simulink model "ClosedLoopSystemAccVar1"  (R2024b)
settings: Solver=FixedStepDiscrete  StartTime=0.0  StopTime=300  MaxStep=0.001  RelTol=1e-5
values from neighbouring files (symbols this model uses):
  A : value not decoded    [eomParameters.sldd]
  B : value not decoded    [eomParameters.sldd]
  b = 0.1    [eomParameters.sldd]
  C : value not decoded    [eomParameters.sldd]
  D : value not decoded    [eomParameters.sldd]
  d : value not decoded    [eomParameters.sldd]
  E : value not decoded    [eomParameters.sldd]
  F : value not decoded    [eomParameters.sldd]
  H : value not decoded    [eomParameters.sldd]
  I : value not decoded    [eomParameters.sldd]
  K : value not decoded    [eomParameters.sldd]
  L_1 : value not decoded    [eomParameters.sldd]
  mu = 0.4    [eomParameters.sldd]
  mu_r = 0.001    [eomParameters.sldd]
undefined symbols (not defined in the file or in its folder): DiscIntNeverNeededParam
libraries: slpidlib x1, simulink x1
settings Model: DataDictionary=eomParameters.sldd  Creator=nilgunozbulbul  LastModifiedBy=nilgunozbulbul
settings SolverCC: InitialStep=0.001

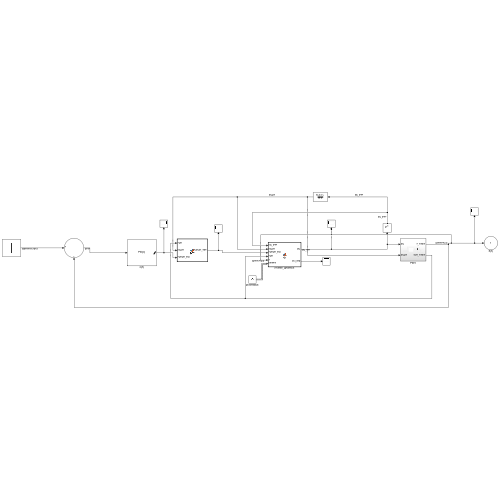
[thumbnail: Simulink's stored preview of the top-level diagram]
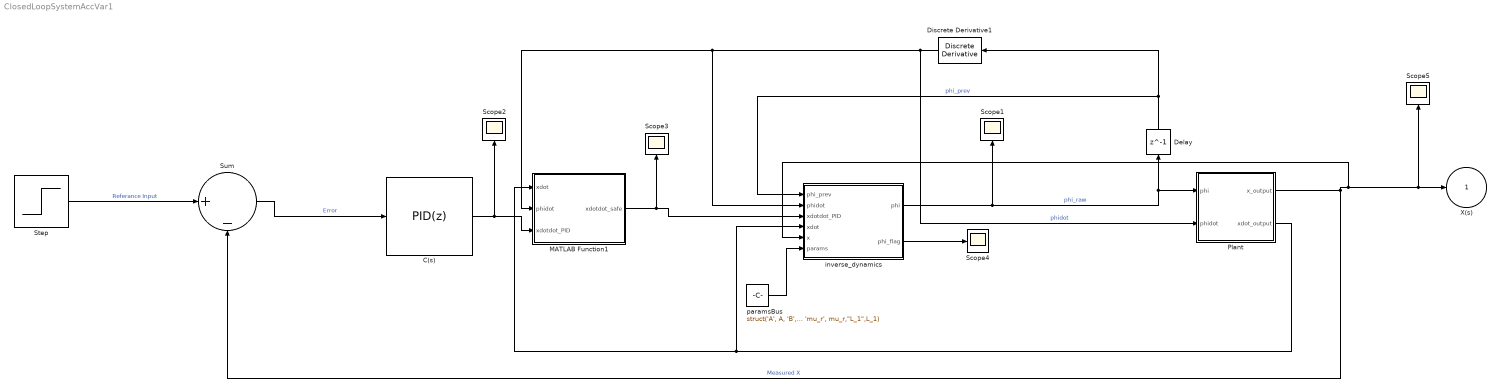
== system ClosedLoopSystemAccVar1 ==
  C(s) : slpidlib/PID Controller  Controller=PID  Form=Parallel  TimeDomain=Discrete-time  UseExternalTs=off  SampleTime=0.05  IntegratorMethod=Forward Euler  FilterMethod=Forward Euler  ControllerParametersSource=internal  P=1  I=1  UseKiTs=off  D=1  UseExternalDerivativeSource=off  N=100  UseFilter=on  TunerSelectOption=Frequency Response Based  InitialConditionSource=internal  InitialConditionForIntegrator=0  InitialConditionForFilter=0  DifferentiatorICPrevScaledInput=0  ExternalReset=none  TrackingMode=off  Kt=1  LimitOutput=on  SatLimitsSource=internal  UpperSaturationLimit=8  LowerSaturationLimit=-8  LinearizeAsGain=off  AntiWindupMode=back-calculation  Kb=1  LimitIntegrator=on  UpperIntegratorSaturationLimit=0.1  LowerIntegratorSaturationLimit=-0.1  POutMin=[]  POutMax=[]  IOutMin=[]  IOutMax=[]  DOutMin=[]  DOutMax=[]  NOutMin=[]  NOutMax=[]  SumOutMin=[]  SumOutMax=[]  SaturationOutMin=[]  SaturationOutMax=[]  PParamMin=[]  PParamMax=[]  IParamMin=[]  IParamMax=[]  DParamMin=[]  DParamMax=[]  NParamMin=[]  NParamMax=[]  KbParamMin=[]  KbParamMax=[]  KtParamMin=[]  KtParamMax=[]  KbOutMin=[]  KbOutMax=[]  KtOutMin=[]  KtOutMax=[]  IntegratorOutMin=[]  IntegratorOutMax=[]  FilterOutMin=[]  FilterOutMax=[]  SumI1OutMin=[]  SumI1OutMax=[]  SumI2OutMin=[]  SumI2OutMax=[]  SumI3OutMin=[]  SumI3OutMax=[]  SumI4OutMin=[]  SumI4OutMax=[]  SumDOutMin=[]  SumDOutMax=[]  DifferentiatorOutMin=[]  DifferentiatorOutMax=[]  FilterDiffOutCoefMin=[]  FilterDiffOutCoefMax=[]  ReciprocalOutMin=[]  ReciprocalOutMax=[]  SumDenOutMin=[]  SumDenOutMax=[]  SumNumOutMin=[]  SumNumOutMax=[]  DivideOutMin=[]  DivideOutMax=[]  UdiffTsProdOutMin=[]  UdiffTsProdOutMax=[]  NTsProdOutMin=[]  NTsProdOutMax=[]  UintegralTsProdOutMin=[]  UintegralTsProdOutMax=[]  UngainTsProdOutMin=[]  UngainTsProdOutMax=[]  ClampingZeroOutDataTypeStr=Inherit: Inherit via back propagation  ClampingZeroOutMin=[]  ClampingZeroOutMax=[]  FilterDenConstantOutDataTypeStr=Inherit: Inherit via back propagation  FilterDenConstantOutMin=[]  FilterDenConstantOutMax=[]  PCopyOutDataTypeStr=Inherit: Inherit via back propagation  PCopyOutMin=[]  PCopyOutMax=[]  NCopyOutDataTypeStr=Inherit: Inherit via back propagation  NCopyOutMin=[]  NCopyOutMax=[]  IntegratorContinuousStateAttributes=''  IntegratorStateMustResolveToSignalObject=off  IntegratorRTWStateStorageClass=Auto  FilterContinuousStateAttributes=''  FilterStateMustResolveToSignalObject=off  FilterRTWStateStorageClass=Auto  ParallelPVariant=InternalParameters  IdealPVariant=Disabled  IVariant=InternalParameters  DVariant=InternalParameters  IntegratorVariant=Discrete  SatVariant=Enabled  AWVariant=BackCalculation  PCopyVariant=Disabled  TRVariant=Disabled  FdbkBlocksVariant=Forward  IdealPFdbkVariant=Disabled  SatFdbkVariant=Disabled  DerivativeFilterVariant=ForwardEulerFilter  NVariant=InternalParameters  NCopyVariant=Disabled  FilterICVariant=InternalICsFilter  IntegratorICVariant=InternalICs  ExternalResetVariant=Disabled  TRSumVariant=Passthrough  SumFdbkVariant=Disabled  SumVariant=Sum_PID  TsampFilterVariant=InternalTs  TsampNgainVariant=Passthrough  TsampIntegralVariant=Disabled_SignalSpec  ExternalSaturationOutDataTypeStr=Inherit: Same as second input  DerivativeSourceVariant=ErrorSignal  PreIntVariant=InternalPreInt
      settings: LibrarySourceBlock=simulink/Discrete/Discrete PID Controller
  Delay : Delay  DelayLength=1  InitialCondition=0  SampleTime=0.05
  Discrete Derivative1 : simulink/Discrete/Discrete Derivative  gainval=1.0  ICPrevScaledInput=0.0  OutMin=[]  OutMax=[]  OutDataType=fixdt(1, 16)  OutScaling=2^-10  DoSatur=off
  MATLAB Function1 : MATLAB Function  TreatAsAtomicUnit=on
  Plant : Subsystem
  Scope{1..5} (5 alike) : Scope
  Step : Step  Time=0  After=0.05  SampleTime=0.05
  Sum : Sum  Inputs=|+-
  inverse_dynamics : MATLAB Function  TreatAsAtomicUnit=on
  paramsBus : Constant  Value="struct('A', A, 'B', B, 'C', C, 'D', D, 'E', E, 'F', F, 'H', H, 'I', I, 'K', K, 'b', b, 'd', d, 'mu', mu, 'mu_r', mu_r,\"L_1\",L_1)"  OutDataTypeStr=Bus: paramsBus
  X(s) : Outport
  wires:
  Plant/1(x_output) -> Scope5/1, X(s)/1, inverse_dynamics/5(x), Sum/2  "Measured X"
  Delay/1 -> inverse_dynamics/1(phi_prev), Discrete Derivative1/1  "phi_prev"
  inverse_dynamics/2(phi_flag) -> Scope4/1
  paramsBus/1 -> inverse_dynamics/6(params)
  Discrete Derivative1/1 -> Plant/2(phidot), MATLAB Function1/2(phidot), inverse_dynamics/2(phidot)  "phidot"
  Plant/2(xdot_output) -> MATLAB Function1/1(xdot), inverse_dynamics/4(xdot)
  Sum/1 -> C(s)/1  "Error"
  inverse_dynamics/1(phi) -> Scope1/1, Delay/1, Plant/1(phi)  "phi_raw"
  C(s)/1 -> Scope2/1, MATLAB Function1/3(xdotdot_PID)
  MATLAB Function1/1(xdotdot_safe) -> Scope3/1, inverse_dynamics/3(xdotdot_PID)
  Step/1 -> Sum/1  "Referance Input"

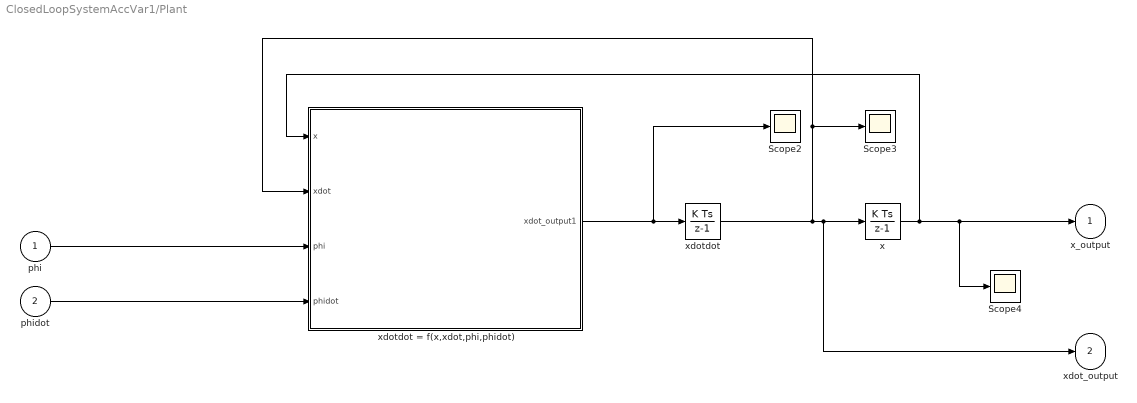
== system ClosedLoopSystemAccVar1/Plant ==
  phi : Inport
  phidot : Inport  Port=2
  Scope2 : Scope
  Scope3 : Scope
  Scope4 : Scope
  x : DiscreteIntegrator  InitialCondition=0.05  SampleTime=0.05  UpperSaturationLimit=+100  LowerSaturationLimit=-100  ICPrevOutput=DiscIntNeverNeededParam  ICPrevScaledInput=DiscIntNeverNeededParam
  xdotdot : DiscreteIntegrator  InitialCondition=0.1  SampleTime=0.05  UpperSaturationLimit=+100  LowerSaturationLimit=-100  ICPrevOutput=DiscIntNeverNeededParam  ICPrevScaledInput=DiscIntNeverNeededParam
  xdotdot = f(x,xdot,phi,phidot) : Subsystem
  x_output : Outport
  xdot_output : Outport  Port=2
  wires:
  x/1 -> xdotdot = f(x,xdot,phi,phidot)/1(x), Scope4/1, x_output/1
  xdotdot = f(x,xdot,phi,phidot)/1(xdot_output1) -> xdotdot/1, Scope2/1
  phi/1 -> xdotdot = f(x,xdot,phi,phidot)/3(phi)
  xdotdot/1 -> Scope3/1, xdotdot = f(x,xdot,phi,phidot)/2(xdot), xdot_output/1, x/1
  phidot/1 -> xdotdot = f(x,xdot,phi,phidot)/4(phidot)

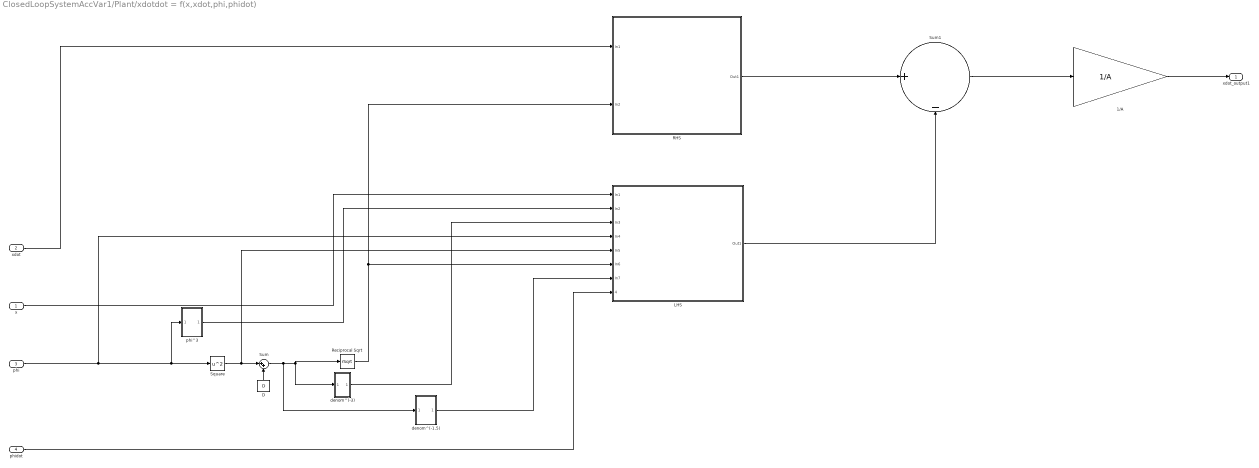
== system ClosedLoopSystemAccVar1/Plant/xdotdot = f(x,xdot,phi,phidot) ==
  x : Inport
  xdot : Inport  Port=2
  phi : Inport  Port=3
  phidot : Inport  Port=4
  1/A : Gain  Gain=1/A
  D : Constant  Value=D
  LHS : Subsystem
  RHS : Subsystem
  Reciprocal Sqrt : Sqrt  Operator=rSqrt
  Square : Math  Operator=square
  Sum : Sum  Inputs=|++
  Sum1 : Sum  Inputs=|+-
  denom^(-1.5) : Subsystem
  denom^(-3) : Subsystem
  phi^3 : Subsystem
  xdot_output1 : Outport
  wires:
  phi/1 -> LHS/4(In4), Square/1, phi^3/1(In1)
  Square/1 -> LHS/5(In5), Sum/1
  D/1 -> Sum/2
  Reciprocal Sqrt/1 -> LHS/6(In6), RHS/2(In2)
  Sum/1 -> Reciprocal Sqrt/1, denom^(-3)/1(In1), denom^(-1.5)/1(In1)
  xdot/1 -> RHS/1(In1)
  x/1 -> LHS/1(In1)
  phi^3/1(Out1) -> LHS/2(In2)
  denom^(-3)/1(Out1) -> LHS/3(In3)
  denom^(-1.5)/1(Out1) -> LHS/7(In7)
  phidot/1 -> LHS/8(4)
  RHS/1(Out1) -> Sum1/1
  LHS/1(Out1) -> Sum1/2
  Sum1/1 -> 1/A/1
  1/A/1 -> xdot_output1/1

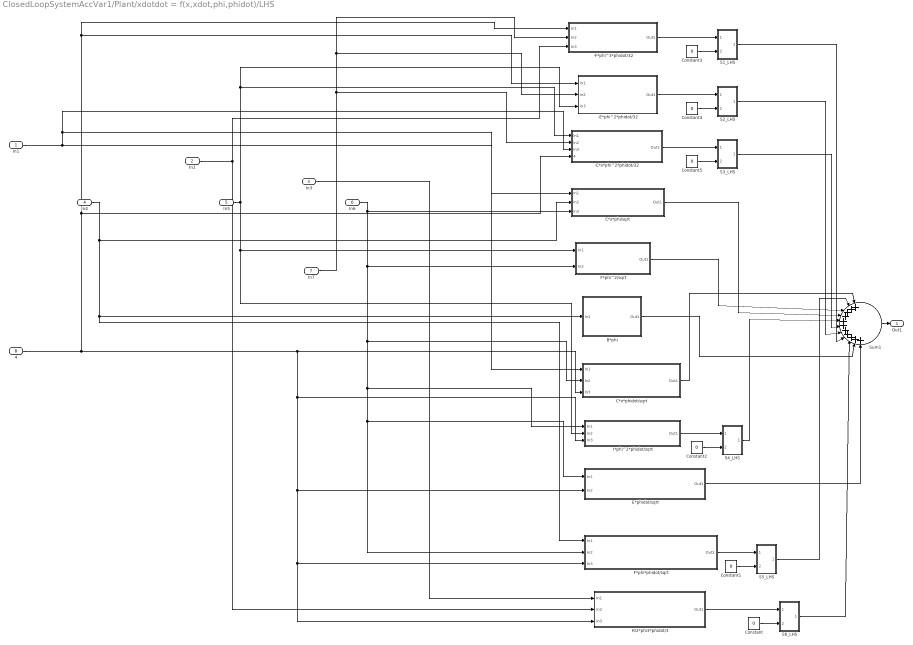
== system ClosedLoopSystemAccVar1/Plant/xdotdot = f(x,xdot,phi,phidot)/LHS ==
  In1 : Inport
  In2 : Inport  Port=2
  In3 : Inport  Port=3
  In4 : Inport  Port=4
  In5 : Inport  Port=5
  In6 : Inport  Port=6
  In7 : Inport  Port=7
  4 : Inport  Port=8
  -C*x*phi^2*phidot/32 : Subsystem
  -E*phi^2*phidot/32 : Subsystem
  -F*phi^3*phidot/32 : Subsystem
  B*phi : Subsystem
  C*x*phi/sqrt : Subsystem
  C*x*phidot/sqrt : Subsystem
  Constant{,1..5} (6 alike) : Constant  Value=0
  E*phidot/sqrt : Subsystem
  F*phi*phidot/sqrt : Subsystem
  F*phi^2/sqrt : Subsystem
  H/2*phi3*phidot/3 : Subsystem
  I*phi^2*phidot/sqrt : Subsystem
  S1_LHS : Subsystem
  S2_LHS : Subsystem
  S3_LHS : Subsystem
  S4_LHS : Subsystem
  S5_LHS : Subsystem
  S6_LHS : Subsystem
  Sum1 : Sum  Inputs=|+++++++++++
  Out1 : Outport
  wires:
  C*x*phi/sqrt/1(Out1) -> Sum1/4
  F*phi^2/sqrt/1(Out1) -> Sum1/3
  C*x*phidot/sqrt/1(Out1) -> Sum1/1
  Sum1/1 -> Out1/1
  In7/1 -> -F*phi^3*phidot/32/2(In2), -E*phi^2*phidot/32/2(In2), -C*x*phi^2*phidot/32/2(In2)
  In5/1 -> F*phi^2/sqrt/1(In1), I*phi^2*phidot/sqrt/2(In2), -E*phi^2*phidot/32/3(In3), -C*x*phi^2*phidot/32/1(In1)
  E*phidot/sqrt/1(Out1) -> Sum1/11
  B*phi/1(Out1) -> Sum1/10
  In2/1 -> H/2*phi3*phidot/3/2(In2), -F*phi^3*phidot/32/3(In3)
  In1/1 -> C*x*phidot/sqrt/1(In1), -C*x*phi^2*phidot/32/3(In3), C*x*phi/sqrt/1(In1)
  In3/1 -> H/2*phi3*phidot/3/1(In1)
  In4/1 -> C*x*phi/sqrt/2(In2), F*phi*phidot/sqrt/1(In1), B*phi/1(In1)
  In6/1 -> F*phi^2/sqrt/2(In2), I*phi^2*phidot/sqrt/1(In1), E*phidot/sqrt/1(In1), F*phi*phidot/sqrt/2(In2), C*x*phidot/sqrt/2(In2), C*x*phi/sqrt/3(In3)
  4/1 -> -F*phi^3*phidot/32/1(In1), -E*phi^2*phidot/32/1(In1), -C*x*phi^2*phidot/32/4(4), F*phi*phidot/sqrt/3(In3), H/2*phi3*phidot/3/3(In3), E*phidot/sqrt/2(In2), I*phi^2*phidot/sqrt/3(In3), C*x*phidot/sqrt/3(In3)
  Constant/1 -> S6_LHS/2(In2)
  H/2*phi3*phidot/3/1(Out1) -> S6_LHS/1(In1)
  S6_LHS/1(Out1) -> Sum1/9
  Constant1/1 -> S5_LHS/2(In2)
  F*phi*phidot/sqrt/1(Out1) -> S5_LHS/1(In1)
  S5_LHS/1(Out1) -> Sum1/2
  Constant2/1 -> S4_LHS/2(In2)
  I*phi^2*phidot/sqrt/1(Out1) -> S4_LHS/1(In1)
  S4_LHS/1(Out1) -> Sum1/5
  Constant3/1 -> S1_LHS/2(In2)
  Constant4/1 -> S2_LHS/2(In2)
  Constant5/1 -> S3_LHS/2(In2)
  -F*phi^3*phidot/32/1(Out1) -> S1_LHS/1(In1)
  -E*phi^2*phidot/32/1(Out1) -> S2_LHS/1(In1)
  -C*x*phi^2*phidot/32/1(Out1) -> S3_LHS/1(In1)
  S3_LHS/1(Out1) -> Sum1/6
  S2_LHS/1(Out1) -> Sum1/7
  S1_LHS/1(Out1) -> Sum1/8

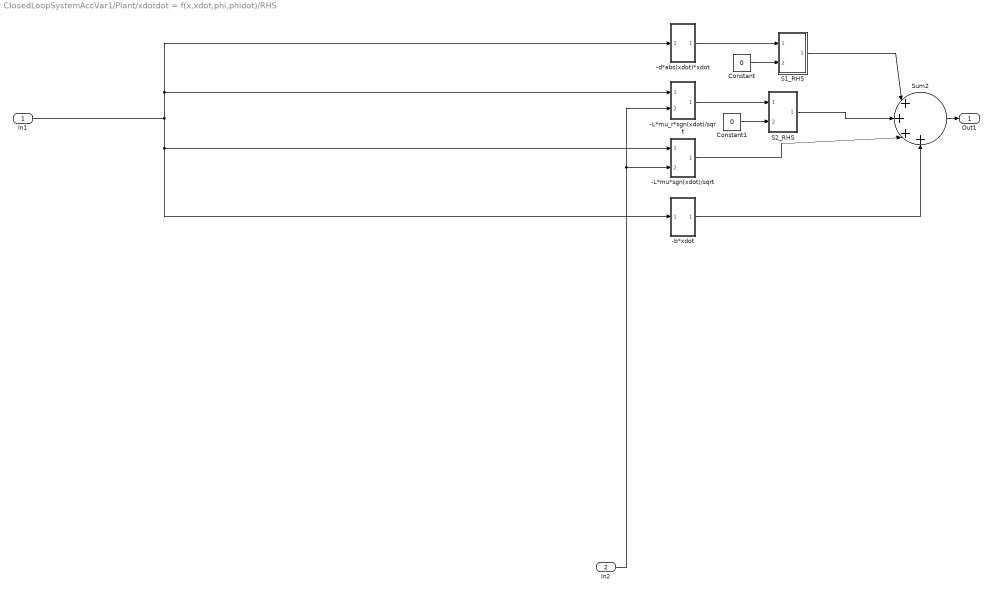
== system ClosedLoopSystemAccVar1/Plant/xdotdot = f(x,xdot,phi,phidot)/RHS ==
  In1 : Inport
  In2 : Inport  Port=2
  -L*mu*sgn(xdot)/sqrt : Subsystem
  -L*mu_r*sgn(xdot)/sqrt : Subsystem
  -b*xdot : Subsystem
  -d*abs(xdot)*xdot : Subsystem
  Constant : Constant  Value=0
  Constant1 : Constant  Value=0
  S1_RHS : Subsystem
  S2_RHS : Subsystem
  Sum2 : Sum  Inputs=|++++
  Out1 : Outport
  wires:
  Sum2/1 -> Out1/1
  -L*mu*sgn(xdot)/sqrt/1(Out1) -> Sum2/3
  -b*xdot/1(Out1) -> Sum2/4
  In1/1 -> -d*abs(xdot)*xdot/1(In1), -L*mu_r*sgn(xdot)/sqrt/1(In1), -b*xdot/1(In1), -L*mu*sgn(xdot)/sqrt/1(In1)
  In2/1 -> -L*mu_r*sgn(xdot)/sqrt/2(In2), -L*mu*sgn(xdot)/sqrt/2(In2)
  Constant/1 -> S1_RHS/2(In2)
  -d*abs(xdot)*xdot/1(Out1) -> S1_RHS/1(In1)
  S1_RHS/1(Out1) -> Sum2/1
  Constant1/1 -> S2_RHS/2(In2)
  -L*mu_r*sgn(xdot)/sqrt/1(Out1) -> S2_RHS/1(In1)
  S2_RHS/1(Out1) -> Sum2/2

== system ClosedLoopSystemAccVar1/Plant/xdotdot = f(x,xdot,phi,phidot)/denom^(-1.5) ==
  In1 : Inport
  3/2 : Constant  Value=-1.5
  Power1 : Math  Operator=pow
  Out1 : Outport
  wires:
  In1/1 -> Power1/1
  Power1/1 -> Out1/1
  3/2/1 -> Power1/2

== system ClosedLoopSystemAccVar1/Plant/xdotdot = f(x,xdot,phi,phidot)/denom^(-3) ==
  In1 : Inport
  3 : Constant  Value=-3
  Power2 : Math  Operator=pow
  Out1 : Outport
  wires:
  Power2/1 -> Out1/1
  In1/1 -> Power2/1
  3/1 -> Power2/2

== system ClosedLoopSystemAccVar1/Plant/xdotdot = f(x,xdot,phi,phidot)/phi^3 ==
  In1 : Inport
  3_ : Constant  Value=3
  Power3 : Math  Operator=pow
  Out1 : Outport
  wires:
  Power3/1 -> Out1/1
  In1/1 -> Power3/1
  3_/1 -> Power3/2

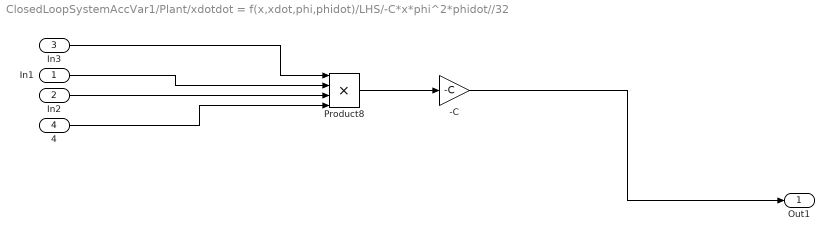
== system ClosedLoopSystemAccVar1/Plant/xdotdot = f(x,xdot,phi,phidot)/LHS/-C*x*phi^2*phidot//32 ==
  In1 : Inport
  In2 : Inport  Port=2
  In3 : Inport  Port=3
  4 : Inport  Port=4
  -C : Gain  Gain=-C
  Product8 : Product  Inputs=4
  Out1 : Outport
  wires:
  -C/1 -> Out1/1
  In2/1 -> Product8/3
  In3/1 -> Product8/1
  In1/1 -> Product8/2
  Product8/1 -> -C/1
  4/1 -> Product8/4

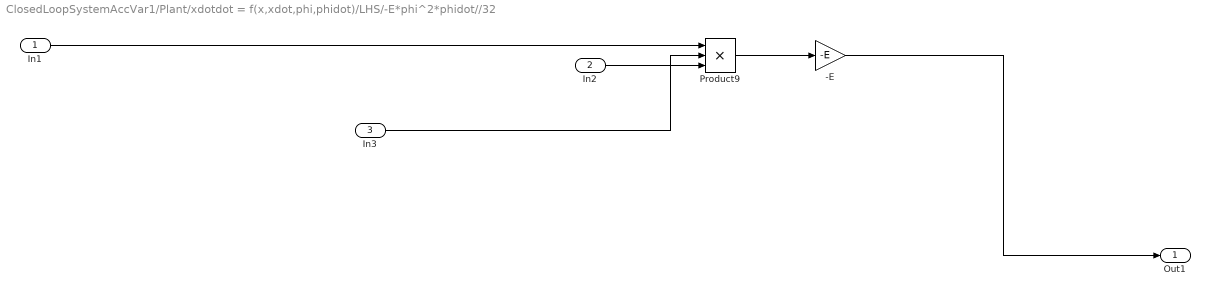
== system ClosedLoopSystemAccVar1/Plant/xdotdot = f(x,xdot,phi,phidot)/LHS/-E*phi^2*phidot//32 ==
  In1 : Inport
  In2 : Inport  Port=2
  In3 : Inport  Port=3
  -E : Gain  Gain=-E
  Product9 : Product  Inputs=3
  Out1 : Outport
  wires:
  -E/1 -> Out1/1
  In2/1 -> Product9/3
  In1/1 -> Product9/1
  In3/1 -> Product9/2
  Product9/1 -> -E/1

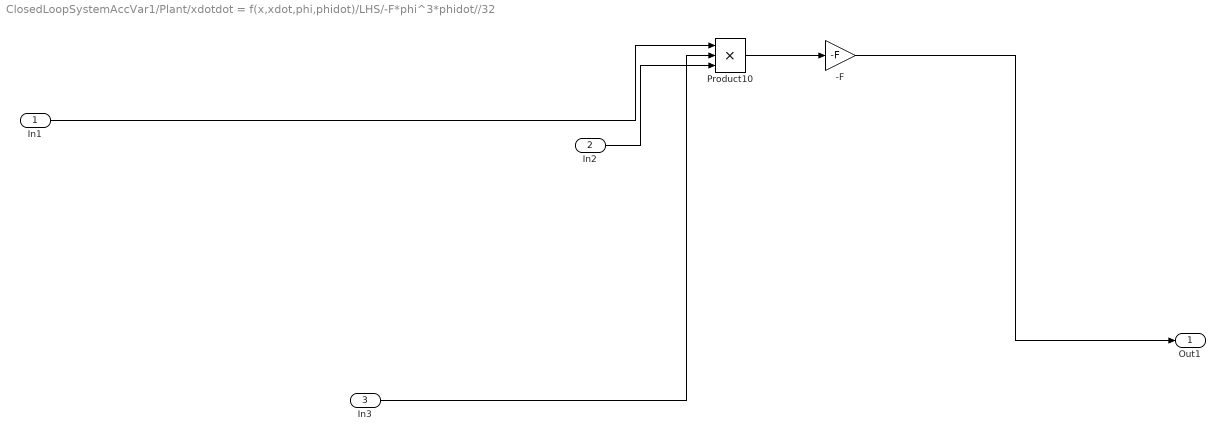
== system ClosedLoopSystemAccVar1/Plant/xdotdot = f(x,xdot,phi,phidot)/LHS/-F*phi^3*phidot//32 ==
  In1 : Inport
  In2 : Inport  Port=2
  In3 : Inport  Port=3
  -F : Gain  Gain=-F
  Product10 : Product  Inputs=3
  Out1 : Outport
  wires:
  In3/1 -> Product10/2
  -F/1 -> Out1/1
  In2/1 -> Product10/3
  In1/1 -> Product10/1
  Product10/1 -> -F/1

== system ClosedLoopSystemAccVar1/Plant/xdotdot = f(x,xdot,phi,phidot)/LHS/B*phi ==
  In1 : Inport
  B : Gain  Gain=B
  Out1 : Outport
  wires:
  In1/1 -> B/1
  B/1 -> Out1/1

== system ClosedLoopSystemAccVar1/Plant/xdotdot = f(x,xdot,phi,phidot)/LHS/C*x*phi//sqrt ==
  In1 : Inport
  In2 : Inport  Port=2
  In3 : Inport  Port=3
  C : Gain  Gain=C
  Product3 : Product  Inputs=3
  Out1 : Outport
  wires:
  In1/1 -> Product3/2
  In3/1 -> Product3/3
  C/1 -> Out1/1
  In2/1 -> Product3/1
  Product3/1 -> C/1

== system ClosedLoopSystemAccVar1/Plant/xdotdot = f(x,xdot,phi,phidot)/LHS/C*x*phidot//sqrt ==
  In1 : Inport
  In2 : Inport  Port=2
  In3 : Inport  Port=3
  C : Gain  Gain=C
  Product : Product  Inputs=3
  Out1 : Outport
  wires:
  In3/1 -> Product/3
  In1/1 -> Product/1
  In2/1 -> Product/2
  C/1 -> Out1/1
  Product/1 -> C/1

== system ClosedLoopSystemAccVar1/Plant/xdotdot = f(x,xdot,phi,phidot)/LHS/E*phidot//sqrt ==
  In1 : Inport
  In2 : Inport  Port=2
  E : Gain  Gain=E
  Product1 : Product
  Out1 : Outport
  wires:
  In2/1 -> Product1/2
  E/1 -> Out1/1
  In1/1 -> Product1/1
  Product1/1 -> E/1

== system ClosedLoopSystemAccVar1/Plant/xdotdot = f(x,xdot,phi,phidot)/LHS/F*phi*phidot//sqrt ==
  In1 : Inport
  In2 : Inport  Port=2
  In3 : Inport  Port=3
  F : Gain  Gain=F
  Product2 : Product  Inputs=3
  Out1 : Outport
  wires:
  F/1 -> Out1/1
  In2/1 -> Product2/2
  In3/1 -> Product2/1
  In1/1 -> Product2/3
  Product2/1 -> F/1

== system ClosedLoopSystemAccVar1/Plant/xdotdot = f(x,xdot,phi,phidot)/LHS/F*phi^2//sqrt ==
  In1 : Inport
  In2 : Inport  Port=2
  F : Gain  Gain=F
  Product4 : Product
  Out1 : Outport
  wires:
  F/1 -> Out1/1
  In1/1 -> Product4/2
  In2/1 -> Product4/1
  Product4/1 -> F/1

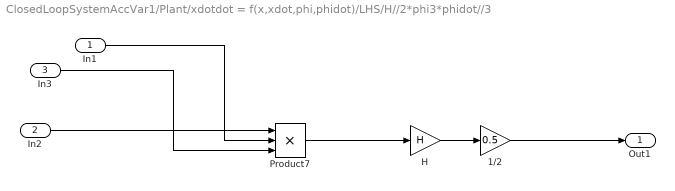
== system ClosedLoopSystemAccVar1/Plant/xdotdot = f(x,xdot,phi,phidot)/LHS/H//2*phi3*phidot//3 ==
  In1 : Inport
  In2 : Inport  Port=2
  In3 : Inport  Port=3
  1/2 : Gain  Gain=0.5
  H : Gain  Gain=H
  Product7 : Product  Inputs=3
  Out1 : Outport
  wires:
  In2/1 -> Product7/1
  In1/1 -> Product7/2
  In3/1 -> Product7/3
  Product7/1 -> H/1
  1/2/1 -> Out1/1
  H/1 -> 1/2/1

== system ClosedLoopSystemAccVar1/Plant/xdotdot = f(x,xdot,phi,phidot)/LHS/I*phi^2*phidot//sqrt ==
  In1 : Inport
  In2 : Inport  Port=2
  In3 : Inport  Port=3
  I : Gain  Gain=I
  Product11 : Product  Inputs=3
  Out1 : Outport
  wires:
  I/1 -> Out1/1
  In3/1 -> Product11/3
  In2/1 -> Product11/2
  In1/1 -> Product11/1
  Product11/1 -> I/1

== system ClosedLoopSystemAccVar1/Plant/xdotdot = f(x,xdot,phi,phidot)/LHS/S1_LHS ==
  In1 : Inport
  In2 : Inport  Port=2
  Constant1 : Constant  Value=0
  Switch : Switch  Criteria=u2 ~= 0  SaturateOnIntegerOverflow=off  InputSameDT=off
  Out1 : Outport
  wires:
  In1/1 -> Switch/1
  Switch/1 -> Out1/1
  In2/1 -> Switch/2
  Constant1/1 -> Switch/3

== system ClosedLoopSystemAccVar1/Plant/xdotdot = f(x,xdot,phi,phidot)/LHS/S2_LHS ==
  In1 : Inport
  In2 : Inport  Port=2
  Constant1 : Constant  Value=0
  Switch : Switch  Criteria=u2 ~= 0  SaturateOnIntegerOverflow=off  InputSameDT=off
  Out1 : Outport
  wires:
  In1/1 -> Switch/1
  Switch/1 -> Out1/1
  In2/1 -> Switch/2
  Constant1/1 -> Switch/3

== system ClosedLoopSystemAccVar1/Plant/xdotdot = f(x,xdot,phi,phidot)/LHS/S3_LHS ==
  In1 : Inport
  In2 : Inport  Port=2
  Constant1 : Constant  Value=0
  Switch : Switch  Criteria=u2 ~= 0  SaturateOnIntegerOverflow=off  InputSameDT=off
  Out1 : Outport
  wires:
  In1/1 -> Switch/1
  Switch/1 -> Out1/1
  In2/1 -> Switch/2
  Constant1/1 -> Switch/3

== system ClosedLoopSystemAccVar1/Plant/xdotdot = f(x,xdot,phi,phidot)/LHS/S4_LHS ==
  In1 : Inport
  In2 : Inport  Port=2
  Constant1 : Constant  Value=0
  Switch : Switch  Criteria=u2 ~= 0  SaturateOnIntegerOverflow=off  InputSameDT=off
  Out1 : Outport
  wires:
  In1/1 -> Switch/1
  Switch/1 -> Out1/1
  In2/1 -> Switch/2
  Constant1/1 -> Switch/3

== system ClosedLoopSystemAccVar1/Plant/xdotdot = f(x,xdot,phi,phidot)/LHS/S5_LHS ==
  In1 : Inport
  In2 : Inport  Port=2
  Constant1 : Constant  Value=0
  Switch : Switch  Criteria=u2 ~= 0  SaturateOnIntegerOverflow=off  InputSameDT=off
  Out1 : Outport
  wires:
  In1/1 -> Switch/1
  Switch/1 -> Out1/1
  In2/1 -> Switch/2
  Constant1/1 -> Switch/3

== system ClosedLoopSystemAccVar1/Plant/xdotdot = f(x,xdot,phi,phidot)/LHS/S6_LHS ==
  In1 : Inport
  In2 : Inport  Port=2
  Constant1 : Constant  Value=0
  Switch : Switch  Criteria=u2 ~= 0  SaturateOnIntegerOverflow=off  InputSameDT=off
  Out1 : Outport
  wires:
  In1/1 -> Switch/1
  Switch/1 -> Out1/1
  In2/1 -> Switch/2
  Constant1/1 -> Switch/3

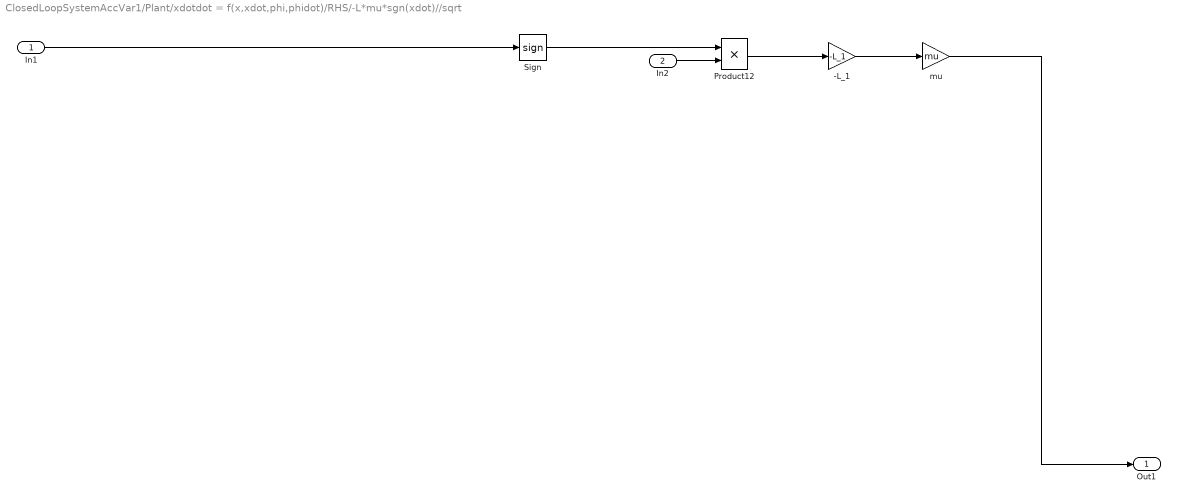
== system ClosedLoopSystemAccVar1/Plant/xdotdot = f(x,xdot,phi,phidot)/RHS/-L*mu*sgn(xdot)//sqrt ==
  In1 : Inport
  In2 : Inport  Port=2
  -L_1 : Gain  Gain=-L_1
  Product12 : Product
  Sign : Signum  ZeroCross=off
  mu : Gain  Gain=mu
  Out1 : Outport
  wires:
  In2/1 -> Product12/2
  Sign/1 -> Product12/1
  In1/1 -> Sign/1
  mu/1 -> Out1/1
  Product12/1 -> -L_1/1
  -L_1/1 -> mu/1

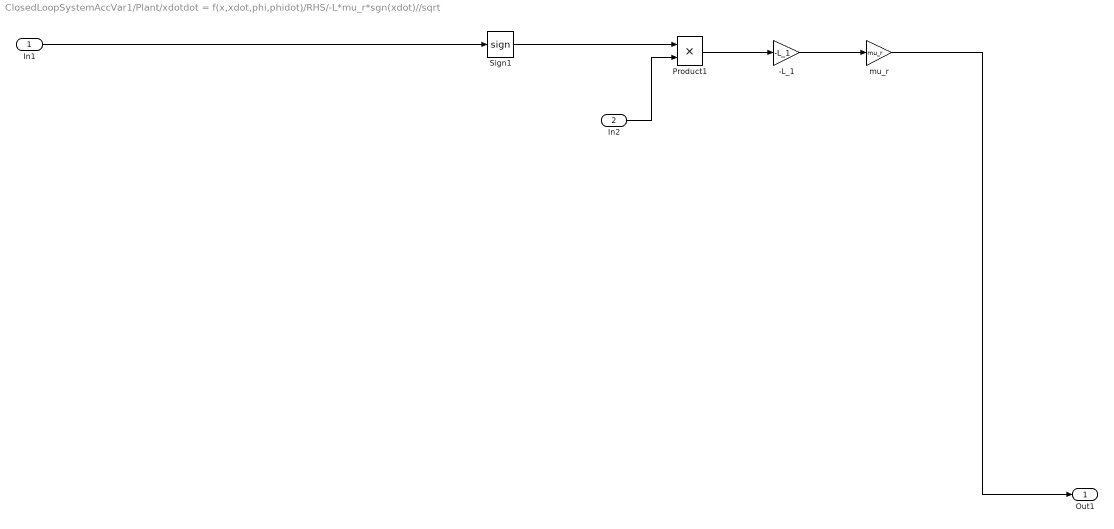
== system ClosedLoopSystemAccVar1/Plant/xdotdot = f(x,xdot,phi,phidot)/RHS/-L*mu_r*sgn(xdot)//sqrt ==
  In1 : Inport
  In2 : Inport  Port=2
  -L_1 : Gain  Gain=-L_1
  Product1 : Product
  Sign1 : Signum  ZeroCross=off
  mu_r : Gain  Gain=mu_r
  Out1 : Outport
  wires:
  Product1/1 -> -L_1/1
  -L_1/1 -> mu_r/1
  Sign1/1 -> Product1/1
  In1/1 -> Sign1/1
  In2/1 -> Product1/2
  mu_r/1 -> Out1/1

== system ClosedLoopSystemAccVar1/Plant/xdotdot = f(x,xdot,phi,phidot)/RHS/-b*xdot ==
  In1 : Inport
  -b : Gain  Gain=-b
  Out1 : Outport
  wires:
  In1/1 -> -b/1
  -b/1 -> Out1/1

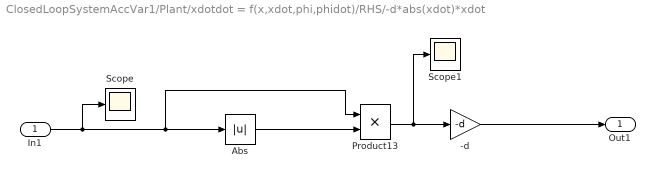
== system ClosedLoopSystemAccVar1/Plant/xdotdot = f(x,xdot,phi,phidot)/RHS/-d*abs(xdot)*xdot ==
  In1 : Inport
  -d : Gain  Gain=-d
  Abs : Abs  ZeroCross=off  SaturateOnIntegerOverflow=off
  Product13 : Product
  Scope : Scope
  Scope1 : Scope
  Out1 : Outport
  wires:
  Product13/1 -> Scope1/1, -d/1
  In1/1 -> Scope/1, Product13/1, Abs/1
  -d/1 -> Out1/1
  Abs/1 -> Product13/2

== system ClosedLoopSystemAccVar1/Plant/xdotdot = f(x,xdot,phi,phidot)/RHS/S1_RHS ==
  In1 : Inport
  In2 : Inport  Port=2
  Constant1 : Constant  Value=0
  Switch : Switch  Criteria=u2 ~= 0  SaturateOnIntegerOverflow=off  InputSameDT=off
  Out1 : Outport
  wires:
  In1/1 -> Switch/1
  Switch/1 -> Out1/1
  In2/1 -> Switch/2
  Constant1/1 -> Switch/3

== system ClosedLoopSystemAccVar1/Plant/xdotdot = f(x,xdot,phi,phidot)/RHS/S2_RHS ==
  In1 : Inport
  In2 : Inport  Port=2
  Constant1 : Constant  Value=0
  Switch : Switch  Criteria=u2 ~= 0  SaturateOnIntegerOverflow=off  InputSameDT=off
  Out1 : Outport
  wires:
  In1/1 -> Switch/1
  Switch/1 -> Out1/1
  In2/1 -> Switch/2
  Constant1/1 -> Switch/3

== matlab function ClosedLoopSystemAccVar1/inverse_dynamics ==
  settings: updateMethod=DISCRETE  sampleTime=0.05
  data: phi_prev input; phidot input; xdotdot_PID input; xdot input; phi output; x input; phi_flag output; params input
function [phi, phi_flag] = fcn(phi_prev, phidot, xdotdot_PID, xdot, x, params)
%#codegen


% --- Bisection & root-finding kısmı ---
Den = params.D;
sqrtDen = sqrt(Den);


f = @(p) ...
      params.A * xdotdot_PID ...
    + params.B * p ...
    + params.C * x * phidot ./ sqrtDen ...
    + params.E * phidot ./ sqrtDen ...
    + params.C * x .* p ./ sqrtDen ...
    + params.F * p.^2 ./ sqrtDen ...
    + params.b * xdot ...
    + params.mu * params.L_1   * sign(xdot) ./ sqrtDen;

a = 0;
b = 0;


% --- Grid scan ile aralık bul ---
phi_min = -180 * pi/180;    % Mutlak limitler (servo limitine uygun)
phi_max = +180 * pi/180;
N_grid = 400;                % Daha fazla = daha hassas
phi_grid = linspace(phi_min, phi_max, N_grid);
f_grid = arrayfun(f, phi_grid);

aralik_bulundu = false;
for i = 1:N_grid-1
    if isfinite(f_grid(i)) && isfinite(f_grid(i+1)) && (f_grid(i) * f_grid(i+1) < 0)
        a = phi_grid(i);
        b = phi_grid(i+1);
        aralik_bulundu = true;
        break;
    end
end

if ~aralik_bulundu
    phi = phi_prev;                % Sonucu koru
    phi_flag = -99;                % Kök yok, gridde işaret değişimi bulunamadı
    phi = mod(phi + pi, 2*pi) - pi;
    return
end

% --- Klasik bisection burada başlar (yalnızca tek aralıkla) ---
max_iter = 80;
tol = 1e-4;
fa = f(a);
fb = f(b);
phi = 0.5 * (a + b);
phi_flag = 1;

for iter = 1:max_iter
    fc = f(phi);

    if ~isfinite(fc)
        phi_flag = -88;
        phi = phi_prev;
        phi = mod(phi + pi, 2*pi) - pi;
        return
    end

    if abs(fc) < tol || abs(b - a) < tol
        phi_flag = 10;
        phi = mod(phi + pi, 2*pi) - pi;
        return
    end

    if fa * fc < 0
        b = phi;
        fb = fc;
    else
        a = phi;
        fa = fc;
    end
    phi = 0.5 * (a + b);
end

phi = mod(phi + pi, 2*pi) - pi;

end

== matlab function ClosedLoopSystemAccVar1/MATLAB Function1 ==
  data: xdotdot_safe output; xdot input; phidot input; xdotdot_PID input
function xdotdot_safe = SCC(xdot, phidot, xdotdot_PID)
% SCC: Safe Set Constraint block
% Girişler:
%   xdot         : Mevcut hız
%   phidot       : Mevcut platform açısal hızı
%   xdotdot_PID  : PID tarafından önerilen ivme (kontrol sinyali)
% Çıkış:
%   xdotdot_safe : Sınırlı (clamp'lı) ivme

    % --- Fit denklemleri ---
    phidot_fit_1 = -0.8093 * xdot - 0.2823 * xdotdot_PID - 0.472;
    phidot_fit_2 =  0.404  - 0.282 * xdotdot_PID - 0.814 * xdot;

    % --- Clamp'lı çıkış (default: PID sinyali) ---
    xdotdot_safe = xdotdot_PID;

    % --- Region 1: xdot < 0 ve phidot < phidot_fit_1 ise clamp yap ---
    if (xdot < 0) && (phidot < phidot_fit_1)
        % Clamp: xdotdot_PID'i, sınırda kök olan değere ayarla
        xdotdot_safe = (phidot + 0.8093 * xdot + 0.472) / (-0.2823);
    end

    % --- Region 2: xdot > 0 ve phidot < phidot_fit_2 ise clamp yap ---
    if (xdot > 0) && (phidot < phidot_fit_2)
        xdotdot_safe = (0.404 - phidot - 0.814 * xdot) / 0.282;
    end

    % --- Ayrıca saturasyon uygulamak istersen burada ekleyebilirsin ---
    % xdotdot_safe = min(max(xdotdot_safe, -8), 8); % Örnek sınırlar

end
